simulink model "elec_linact_implementation"  (R2016a)
settings: Solver=ode23t  StartTime=0.0  StopTime=6  MaxStep=1e-2  RelTol=1e-3  AbsTol=1e-3
PostLoadFcn:
  | pwm_choice=1; % Variant control variable for PWM & H-Bridge subsystem
libraries: fl_lib x109, ee_lib x35, nesl_utility x16, fl_ps_legacy_lib x1, simulink x1
(part 1 of 2)
Description:
  | Linear Electric Actuator (Implementation Model)
  | 
  | This example shows a detailed implementation model of a controlled linear
  | actuator. The actuator consists of a DC motor driving a worm gear which in
  | turn drives a lead screw to produce linear motion. The model includes
  | quantization effects of the Hall-effect sensor and the implementation of the
  | control in analog electronics. Optionally, the PWM switching waveforms of
  | the PWM & H-Bridge subsystem can be included by right clicking on the
  | block and selecting Variant->Override using->pwm_choice==2. To simulate
  | with the actual semiconductor switching devices, select Variant->Override
  | using->pwm_choice==3. The model will run slowly with these options due
  | to the 10kHz switching and/or added component detail, but is useful for
  | validation of the system-averaged mode.
  | 
  | 
  | 
  | 
  | 
  | 
  | Copyright 2008-2016 The MathWorks, Inc.
settings Model: FPTRunName=Active  ExtModeAutoUpdateStatusClock=off  Creator=MathWorks  LastModifiedBy=Alireza
settings SolverCC: MaxConsecutiveMinStep=250  ZeroCrossControl=EnableAll
settings DataIOCC: LimitDataPoints=on  SaveFormat=Array  SignalLoggingSaveFormat=ModelDataLogs
settings OptimizationCC: ExpressionDepthLimit=2147483647  InitFltsAndDblsToZero=on
settings DebuggingCC: SaveWithParameterizedLinksMsg=none  UnderspecifiedInitializationDetection=Classic  MergeDetectMultiDrivingBlocksExec=none  SignalResolutionControl=TryResolveAllWithWarning  SolverPrmCheckMsg=warning  FcnCallInpInsideContextMsg=EnableAllAsWarning  StateNameClashWarn=warning
settings HardwareCC: ProdBitPerPointer=32  ProdLargestAtomicFloat=None  ProdIntDivRoundTo=Undefined  ProdEndianess=Unspecified  ProdWordSize=32  ProdHWDeviceType=32-bit Generic
settings ModelReferenceCC: PropagateSignalLabelsOutOfModel=off
settings GRTTargetCC: TargetFcnLib=ansi_tfl_tmw.mat  CombineOutputUpdateFcns=off  GRTInterface=on
settings ConfigComp: CovSFcnEnable=off
settings SimscapeCC: SimscapeNormalizeSystem=off

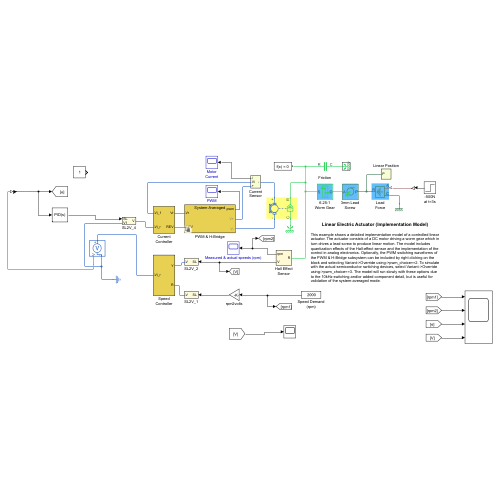
[thumbnail: Simulink's stored preview of the top-level diagram]
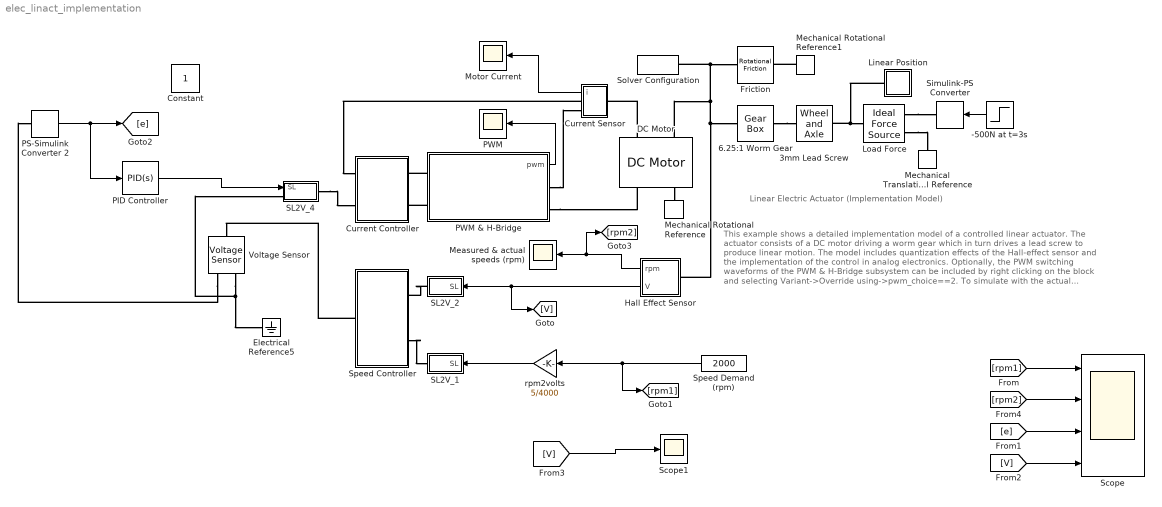
== system elec_linact_implementation ==
  note: Linear Electric Actuator (Implementation Model)
  note: This example shows a detailed implementation model of a controlled linear
      | actuator. The actuator consists of a DC motor driving a worm gear which in
      | turn drives a lead screw to produce linear motion. The model includes
      | quantization effects of the Hall-effect sensor and the implementation of the
      | control in analog electronics. Optionally, the PWM switching waveforms of
      | the PWM & H-Bridge subsystem can be included by right clicking on the
      | block and selecting Variant->Override using->pwm_choice==2. To simulate
      | with the actual semiconductor switching devices, select Variant->Override
      | using->pwm_choice==3. The model will run slowly with these options due
      | to the 10kHz switching and/or added component detail, but is useful for
      | validation of the system-averaged mode.
  -500N at t=3s : Step  Time=3  After=0  SampleTime=0
  3mm Lead Screw : fl_lib/Mechanical/Mechanisms/Wheel and Axle  R=3e-3/(2*pi) m  or=1  t_specify=off  t_priority=High  t=0 N*m  t_nominal_specify=off  t_nominal_unit=N*m  t_nominal_value=1  f_specify=off  f_priority=High  f=0 N  f_nominal_specify=off  f_nominal_unit=N  f_nominal_value=1
  6.25:1 Worm Gear : fl_lib/Mechanical/Mechanisms/Gear Box  ratio=6.25  t_in_specify=off  t_in_priority=High  t_in=0 N*m  t_in_nominal_specify=off  t_in_nominal_unit=N*m  t_in_nominal_value=1  t_out_specify=off  t_out_priority=High  t_out=0 N*m  t_out_nominal_specify=off  t_out_nominal_unit=N*m  t_out_nominal_value=1
  Constant : Constant
  Current Controller : Subsystem
  Current Sensor : Subsystem
  DC Motor : ee_lib/Electromechanical/Brushed Motors/DC Motor  field_option=ee.enum.field_option.pm  Rf=100 Ohm  Lf=1 H  Laf=0.15 H  If0=0 A  parameterization=1  Ra=4.8 Ohm  La=1600e-6 H  emf_or_torque=2  Kv=0.0637 V/rpm  Ki=0.066 N*m/A  T_stall=3e-3*4000/(2*pi*6.25) N*m  w_max=3250 rpm  w_rated=2375 rpm  P_rated=19 W  V_rated=24 V  lam_param=1  i_noload=0 A  V_i_noload=1.5 V  J=2.5e-5 kg*m^2  lam=1e-08 N*m/(rad/s)  speed0=0 rpm  enable_fault_armature=simscape.enum.onoff.off  rev_faulted=1 / 3  G_faulted_armature=1e-5 S  fault_trigger_armature=ee.enum.faults.faultTrigger.temporal  t_fault_armature=1 s  max_permissible_current_armature=inf A  t_fail_on_current_armature=1 s  enable_fault_field=simscape.enum.onoff.off  G_faulted_field=1e-5 S  fault_trigger_field=ee.enum.faults.faultTrigger.temporal  t_fault_field=1 s  max_permissible_current_field=inf A  t_fail_on_current_field=1 s  fault_action=simscape.enum.assert.action.none  alpha=3.93e-3 1/K  Tmeas=25 degC  thermal_mass=100 J/K  initial_temperature=25 degC
  Electrical Reference5 : fl_lib/Electrical/Electrical Elements/Electrical Reference
  Friction : fl_lib/Mechanical/Rotational Elements/Rotational Friction  brkwy_trq=0.022 N*m  brkwy_vel=0.03347 rad/s  Col_trq=0.022 N*m  visc_coef=0 N*m/(rad/s)  w_specify=off  w_priority=High  w=0 rad/s  w_nominal_specify=off  w_nominal_unit=rad/s  w_nominal_value=1  t_specify=off  t_priority=High  t=0 N*m  t_nominal_specify=off  t_nominal_unit=N*m  t_nominal_value=1
  Hall Effect Sensor : Subsystem
  Linear Position : Subsystem
  Load Force : fl_lib/Mechanical/Mechanical Sources/Ideal Force Source
  Measured & actual speeds (rpm) : Scope
  Mechanical Rotational Reference : fl_lib/Mechanical/Rotational Elements/Mechanical Rotational Reference
  Mechanical Rotational Reference1 : fl_lib/Mechanical/Rotational Elements/Mechanical Rotational Reference
  Mechanical Translational Reference : fl_lib/Mechanical/Translational Elements/Mechanical Translational Reference
  Motor Current : Scope
  PID Controller : simulink/Continuous/PID Controller  Controller=PID  Form=Parallel  TimeDomain=Continuous-time  SampleTime=-1  IntegratorMethod=Forward Euler  ControllerParametersSource=internal  P=1.8  I=18  D=0  N=100  UseFilter=on  InitialConditionSource=internal  InitialConditionForIntegrator=0  InitialConditionForFilter=0  DifferentiatorICPrevScaledInput=0  ExternalReset=none  TrackingMode=off  Kt=1  LimitOutput=off  UpperSaturationLimit=inf  LowerSaturationLimit=-inf  LinearizeAsGain=on  AntiWindupMode=none  Kb=1  POutMin=[]  POutMax=[]  IOutMin=[]  IOutMax=[]  DOutMin=[]  DOutMax=[]  NOutMin=[]  NOutMax=[]  SumOutMin=[]  SumOutMax=[]  SaturationOutMin=[]  SaturationOutMax=[]  PParamMin=[]  PParamMax=[]  IParamMin=[]  IParamMax=[]  DParamMin=[]  DParamMax=[]  NParamMin=[]  NParamMax=[]  KbParamMin=[]  KbParamMax=[]  KtParamMin=[]  KtParamMax=[]  KbOutMin=[]  KbOutMax=[]  KtOutMin=[]  KtOutMax=[]  IntegratorOutMin=[]  IntegratorOutMax=[]  FilterOutMin=[]  FilterOutMax=[]  SumI1OutMin=[]  SumI1OutMax=[]  SumI2OutMin=[]  SumI2OutMax=[]  SumI3OutMin=[]  SumI3OutMax=[]  SumDOutMin=[]  SumDOutMax=[]  DifferentiatorOutMin=[]  DifferentiatorOutMax=[]  IntegratorContinuousStateAttributes=''  IntegratorStateMustResolveToSignalObject=off  IntegratorRTWStateStorageClass=Auto  FilterContinuousStateAttributes=''  FilterStateMustResolveToSignalObject=off  FilterRTWStateStorageClass=Auto
  PS-Simulink Converter 2 : nesl_utility/PS-Simulink Converter  PhysicalDomain=network_engine_domain  SubClassName=ps_output  LeftPortType=input  RightPortType=output  PseudoPeriodic=off  Frequencies=[]  VectorFormat=1-D array  Unit=V  AffineConversion=off
  PWM : Scope
  PWM & H-Bridge : Subsystem  Variant=on  OverrideUsingVariant=pwm_choice==1
      settings: AttributesFormatString=%<BlockChoice>
  SL2V_1 : Subsystem
  SL2V_2 : Subsystem
  SL2V_4 : Subsystem
  Scope : Scope  NumInputPorts=4
  Scope1 : Scope
  Simulink-PS Converter : nesl_utility/Simulink-PS Converter  PhysicalDomain=network_engine_domain  SubClassName=ps_input  LeftPortType=input  RightPortType=output  PseudoPeriodic=off  Frequencies=[]  NoiseDistribution=none  NoiseParameters=[]  Unit=N  AffineConversion=off  FilteringAndDerivatives=zero  SimscapeFilterOrder=1  InputFilterTimeConstant=.001  UdotUserProvided=0
  Solver Configuration : nesl_utility/Solver Configuration  PhysicalDomain=network_engine_domain  SubClassName=solver  LeftPortType=input  RightPortType=generic  Tones=[]  Harmonics=[]  SimulateNoise=off  Profile=off  UseLocalSampling=off  EnableSwitchedLinearOptims=on  FrequencyDomain=off  UseCCode=off  RelTol=0.001  AbsTol=1e-06  MinStep=1e-09  ToWorkspace=off  RevertToSquareIcSolve=off  NumHomotopyIterations=100  PhasorMode=off  PhasorModeNumHarmonics=1  IndexReductionMethod=DerivativeReplacement  DoDC=off  ResidualTolerance=1e-9  UseLocalSolver=off  LocalSolverChoice=NE_BACKWARD_EULER_ADVANCER  LocalSolverSampleTime=.001  DoFixedCost=off  MaxNonlinIter=3  MaxModeIter=2  ComputeImpulses=off  ImpulseIterations=2  LinearAlgebra=Sparse  LinearAlgebraNumThread=0  EquationFormulation=NE_TIME_EF  DelaysMemoryBudget=1024  AutomaticFiltering=on  FilteringTimeConstant=0.001  PartitionStorageMethod=AS_NEEDED  PartitionMemoryBudget=1024  PartitionMethod=FAST
  Speed Controller : Subsystem
  Speed Demand (rpm) : Constant  Value=2000
  Voltage Sensor : fl_lib/Electrical/Electrical Sensors/Voltage Sensor
  rpm2volts : Gain  Gain=5/4000
  wires:
  -500N at t=3s/1 -> Simulink-PS Converter/1
  rpm2volts/1 -> SL2V_1/1(SL)
  Hall Effect Sensor/2(V) -> [V], SL2V_2/1(SL)
  Hall Effect Sensor/1(rpm) -> [rpm2], Measured & actual speeds (rpm)/1
  Current Sensor/1(i) -> Motor Current/1
  PWM & H-Bridge/1(pwm) -> PWM/1
  PID Controller/1 -> SL2V_4/1(SL)
  PS-Simulink Converter 2/1 -> [e], PID Controller/1
  Speed Demand (rpm)/1 -> rpm2volts/1, [rpm1]
  [rpm1] -> Scope/1
  [rpm2] -> Scope/2
  [e] -> Scope/3
  [V] -> Scope/4
  [V] -> Scope1/1
  connections:
  DC Motor/RConn2 -- Mechanical Rotational Reference/LConn1
  6.25:1 Worm Gear/RConn1 -- 3mm Lead Screw/LConn1
  Linear Position/LConn1 -- Load Force/LConn1 -- 3mm Lead Screw/RConn1
  Load Force/RConn2 -- Mechanical Translational Reference/LConn1
  Load Force/RConn1 -- Simulink-PS Converter/RConn1
  Hall Effect Sensor/LConn1 -- DC Motor/LConn2 -- Solver Configuration/RConn1 -- Friction/LConn1 -- 6.25:1 Worm Gear/LConn1
  PWM & H-Bridge/RConn1 -- Current Sensor/RConn2
  DC Motor/LConn1 -- Current Sensor/LConn1
  PWM & H-Bridge/LConn1 -- Current Controller/RConn1
  PWM & H-Bridge/LConn2 -- Current Controller/RConn2
  Mechanical Rotational Reference1/LConn1 -- Friction/RConn1
  Speed Controller/LConn2 -- SL2V_1/RConn1
  Current Sensor/RConn1 -- Current Controller/LConn1
  SL2V_2/RConn1 -- Speed Controller/LConn1
  PWM & H-Bridge/RConn2 -- DC Motor/RConn1
  Voltage Sensor/RConn2 -- SL2V_4/LConn1 -- Electrical Reference5/LConn1
  Speed Controller/RConn1 -- Voltage Sensor/LConn1
  SL2V_4/RConn1 -- Current Controller/LConn2
  Voltage Sensor/RConn1 -- PS-Simulink Converter 2/LConn1

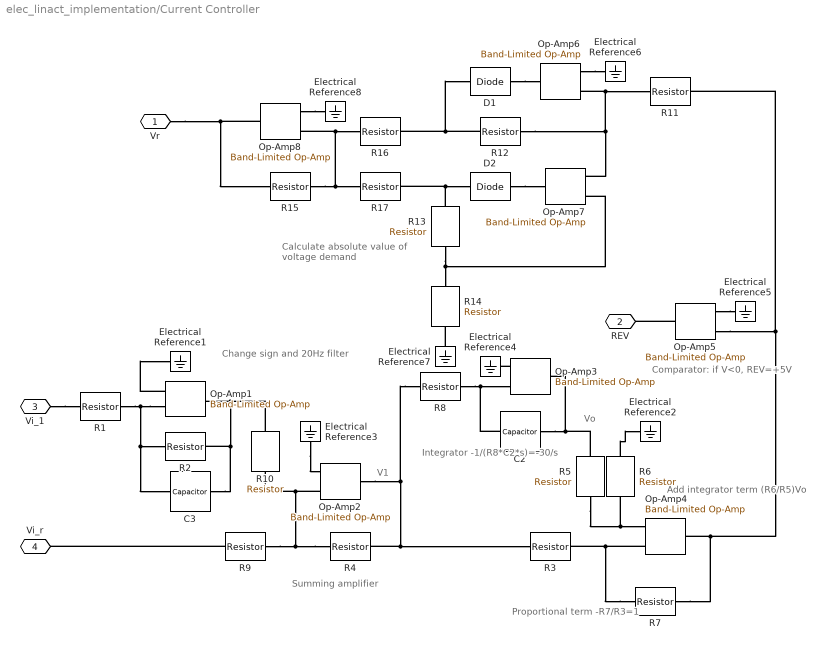
== system elec_linact_implementation/Current Controller ==
  note: Summing
      | amplifier
  note: Integrator
      | -1/(R8*C2*s)=-30/s
  note: Proportional
      | term -R7/R3=1
  note: Add integrator
      | term (R6/R5)Vo
  note: Vo
  note: V1
  note: Change sign
      | and 20Hz filter
  note: Comparator: if
      | V<0, REV=+5V
  note: Calculate absolute value
      | of voltage demand
  C2 : fl_lib/Electrical/Electrical Elements/Capacitor  c=10 uF  r=0.1 Ohm  g=0 1/Ohm  i_specify=off  i_priority=High  i=0 A  i_nominal_specify=off  i_nominal_unit=A  i_nominal_value=1  v_specify=off  v_priority=High  v=0 V  v_nominal_specify=off  v_nominal_unit=V  v_nominal_value=1  vc_specify=on  vc_priority=High  vc=0 V  vc_nominal_specify=off  vc_nominal_unit=V  vc_nominal_value=1
  C3 : fl_lib/Electrical/Electrical Elements/Capacitor  c=0.8 uF  r=0.1 Ohm  g=0 1/Ohm  i_specify=off  i_priority=High  i=0 A  i_nominal_specify=off  i_nominal_unit=A  i_nominal_value=1  v_specify=off  v_priority=High  v=0 V  v_nominal_specify=off  v_nominal_unit=V  v_nominal_value=1  vc_specify=on  vc_priority=High  vc=0 V  vc_nominal_specify=off  vc_nominal_unit=V  vc_nominal_value=1
  D1 : ee_lib/Semiconductors & Converters/Diode  ModelType=ee.enum.diode.modelType.pwl  TableType=ee.enum.diode.tableType.IfMat  IfMat=[.07, .12, .19, 1.75, 4.24, 7.32, 11.2; .16, .3, .72, 2.14, 5.02, 8.35, 13.12] A  VfMat=[.9, 1.15, 1.25, 1.5, 1.75, 2.17, 2.6, 2.85; .58, .68, .75, 1.1, 1.38, 1.77, 2.27, 2.7] V  TjVec=[25, 125] degC  VfVec=[.5, .7, .9, 1.3, 1.7, 2.1, 2.5] V  IfVec=[.1, .2, .5, 1, 2, 4, 7, 10] A  Vf=0.6 V  Ron=0.3 Ohm  Goff=1e-08 1/Ohm  prmExp=1  I12="[  0.07 1.5 ] A"  V12="[  0.7 0.8 ] V"  RS=0 Ohm  Tmeas=298.15 K  IS=1e-14 A  ec=1  I1=0.0137 A  V1=0.6 V  N_series=1  N_parallel=1  Rz=0.3 Ohm  BV=inf V  C_param=1  CJ=5 pF  CJ0=50 pF  Vvec="[  0.1 10 100 ] V"  Cvec="[  3.5 1 0.4 ] pF"  VJ=1 V  Mgrad=0.5  FC=0.5  Q_param=ee.enum.diode.recoveryParam.off  iRM=-7.15 A  iF=4 A  didt=-750 A/us  trr_factor=3  trr=115 ns  Qrr=1500 s*uA  Vr=-600 V  Ls=150 nH  Erec=0.03 J  TT=50 ns  tau=100 ns  T_param=1  Tdevice=25 degC  I1_T2=0.245 A  V1_T2=0.5 V  IS_T2=1.25e-7 A  Tmeas2=125 degC  XTI_param=1  XTI=3  EG_param=1  EG=1.11 eV  dBVdT=0 V/K  enable_faults=simscape.enum.onoff.off  fault_action=simscape.enum.assert.action.none  fault_types=ee.enum.diode.faults.open  tau_fault=1e-3 s  IfMat_faulted=[.07, .12, .19, 1.75, 4.24, 7.32, 11.2; .16, .3, .72, 2.14, 4.02, 6.35, 9.12] A  VfMat_faulted=[.9, 1.15, 1.25, 1.5, 1.75, 2.17, 2.6, 2.85; .58, .68, .75, 1.1, 1.38, 1.77, 2.27, 2.7] V  VfVec_faulted=[.5, .7, .9, 1.3, 1.7, 2.1, 2.5] V  IfVec_faulted=[.1, .2, .5, 1, 2, 4, 7, 10] A  Ropen_faulted=1000 Ohm  Gshort_faulted=1000 1/Ohm  Vf_faulted=0.6 V  Ron_faulted=0.3 Ohm  Goff_faulted=1e-8 S  I12_faulted=[.0137, .545] A  V12_faulted=[.6, .7] V  IS_faulted=1e-12 A  ec_faulted=1  I1_faulted=0.0137 A  V1_faulted=0.6 V  RS_faulted=0 Ohm  Rz_faulted=0.3 Ohm  BV_faulted=inf V  Cscale_faulted=100  enable_temporal_fault=simscape.enum.onoff.off  t_fault=inf s  enable_behavioral_fault=simscape.enum.onoff.off  max_permissible_voltage=inf V  n_fail_on_voltage=1  max_permissible_current=inf A  t_fail_on_current=1 s  max_permissible_dVdt=inf V/s  enable_fault_input=simscape.enum.onoff.off  i_specify=off  i_priority=None  i=0 A  i_nominal_specify=off  i_nominal_unit=A  i_nominal_value=1  v_specify=off  v_priority=None  v=0 V  v_nominal_specify=off  v_nominal_unit=V  v_nominal_value=1  i_diode_specify=off  i_diode_priority=None  i_diode=0 A  i_diode_nominal_specify=off  i_diode_nominal_unit=A  i_diode_nominal_value=1  v_diode_specify=off  v_diode_priority=None  v_diode=0 V  v_diode_nominal_specify=off  v_diode_nominal_unit=V  v_diode_nominal_value=1  i_capacitor_specify=off  i_capacitor_priority=None  i_capacitor=0 A  i_capacitor_nominal_specify=off  i_capacitor_nominal_unit=A  i_capacitor_nominal_value=1  v_capacitor_specify=off  v_capacitor_priority=None  v_capacitor=0 V  v_capacitor_nominal_specify=off  v_capacitor_nominal_unit=V  v_capacitor_nominal_value=1  power_dissipated_specify=off  power_dissipated_priority=None  power_dissipated=0 W  power_dissipated_nominal_specify=off  power_dissipated_nominal_unit=W  power_dissipated_nominal_value=1  max_permissible_temperature=inf K  t_fail_on_temperature=1 s  thermal_network_parameterization=ee.enum.thermalNetworkTopology.junctionCase  Rth=[0, 10] K/W  Rth_Cauer=[1, 3, 10] K/W  Rth_Foster=[4, 6] K/W  thermal_mass_parameterization=ee.enum.thermalNetwork.timeconstant  thermal_mass=[0, 1] J/K  thermal_mass_Cauer=[.1, .3, 1] J/K  thermal_mass_Foster=[1.5, 3] J/K  thermal_time_constant=[0, 10] s  thermal_time_constant_Cauer=[1, 3, 10] s  thermal_time_constant_Foster=[6, 18] s  thermal_mass_initial_temperatures=[25, 25] degC  thermal_mass_initial_temperatures_Cauer=[25, 25, 25] degC  steadyState_Foster=simscape.enum.onoff.on  Tvec_initial_Foster=[25, 25, 25, 25] degC
  D2 : ee_lib/Semiconductors & Converters/Diode  ModelType=ee.enum.diode.modelType.pwl  TableType=ee.enum.diode.tableType.IfMat  IfMat=[.07, .12, .19, 1.75, 4.24, 7.32, 11.2; .16, .3, .72, 2.14, 5.02, 8.35, 13.12] A  VfMat=[.9, 1.15, 1.25, 1.5, 1.75, 2.17, 2.6, 2.85; .58, .68, .75, 1.1, 1.38, 1.77, 2.27, 2.7] V  TjVec=[25, 125] degC  VfVec=[.5, .7, .9, 1.3, 1.7, 2.1, 2.5] V  IfVec=[.1, .2, .5, 1, 2, 4, 7, 10] A  Vf=0.6 V  Ron=0.3 Ohm  Goff=1e-08 1/Ohm  prmExp=1  I12="[  0.07 1.5 ] A"  V12="[  0.7 0.8 ] V"  RS=0 Ohm  Tmeas=298.15 K  IS=1e-14 A  ec=1  I1=0.0137 A  V1=0.6 V  N_series=1  N_parallel=1  Rz=0.3 Ohm  BV=inf V  C_param=1  CJ=5 pF  CJ0=50 pF  Vvec="[  0.1 10 100 ] V"  Cvec="[  3.5 1 0.4 ] pF"  VJ=1 V  Mgrad=0.5  FC=0.5  Q_param=ee.enum.diode.recoveryParam.off  iRM=-7.15 A  iF=4 A  didt=-750 A/us  trr_factor=3  trr=115 ns  Qrr=1500 s*uA  Vr=-600 V  Ls=150 nH  Erec=0.03 J  TT=50 ns  tau=100 ns  T_param=1  Tdevice=25 degC  I1_T2=0.245 A  V1_T2=0.5 V  IS_T2=1.25e-7 A  Tmeas2=125 degC  XTI_param=1  XTI=3  EG_param=1  EG=1.11 eV  dBVdT=0 V/K  enable_faults=simscape.enum.onoff.off  fault_action=simscape.enum.assert.action.none  fault_types=ee.enum.diode.faults.open  tau_fault=1e-3 s  IfMat_faulted=[.07, .12, .19, 1.75, 4.24, 7.32, 11.2; .16, .3, .72, 2.14, 4.02, 6.35, 9.12] A  VfMat_faulted=[.9, 1.15, 1.25, 1.5, 1.75, 2.17, 2.6, 2.85; .58, .68, .75, 1.1, 1.38, 1.77, 2.27, 2.7] V  VfVec_faulted=[.5, .7, .9, 1.3, 1.7, 2.1, 2.5] V  IfVec_faulted=[.1, .2, .5, 1, 2, 4, 7, 10] A  Ropen_faulted=1000 Ohm  Gshort_faulted=1000 1/Ohm  Vf_faulted=0.6 V  Ron_faulted=0.3 Ohm  Goff_faulted=1e-8 S  I12_faulted=[.0137, .545] A  V12_faulted=[.6, .7] V  IS_faulted=1e-12 A  ec_faulted=1  I1_faulted=0.0137 A  V1_faulted=0.6 V  RS_faulted=0 Ohm  Rz_faulted=0.3 Ohm  BV_faulted=inf V  Cscale_faulted=100  enable_temporal_fault=simscape.enum.onoff.off  t_fault=inf s  enable_behavioral_fault=simscape.enum.onoff.off  max_permissible_voltage=inf V  n_fail_on_voltage=1  max_permissible_current=inf A  t_fail_on_current=1 s  max_permissible_dVdt=inf V/s  enable_fault_input=simscape.enum.onoff.off  i_specify=off  i_priority=None  i=0 A  i_nominal_specify=off  i_nominal_unit=A  i_nominal_value=1  v_specify=off  v_priority=None  v=0 V  v_nominal_specify=off  v_nominal_unit=V  v_nominal_value=1  i_diode_specify=off  i_diode_priority=None  i_diode=0 A  i_diode_nominal_specify=off  i_diode_nominal_unit=A  i_diode_nominal_value=1  v_diode_specify=off  v_diode_priority=None  v_diode=0 V  v_diode_nominal_specify=off  v_diode_nominal_unit=V  v_diode_nominal_value=1  i_capacitor_specify=off  i_capacitor_priority=None  i_capacitor=0 A  i_capacitor_nominal_specify=off  i_capacitor_nominal_unit=A  i_capacitor_nominal_value=1  v_capacitor_specify=off  v_capacitor_priority=None  v_capacitor=0 V  v_capacitor_nominal_specify=off  v_capacitor_nominal_unit=V  v_capacitor_nominal_value=1  power_dissipated_specify=off  power_dissipated_priority=None  power_dissipated=0 W  power_dissipated_nominal_specify=off  power_dissipated_nominal_unit=W  power_dissipated_nominal_value=1  max_permissible_temperature=inf K  t_fail_on_temperature=1 s  thermal_network_parameterization=ee.enum.thermalNetworkTopology.junctionCase  Rth=[0, 10] K/W  Rth_Cauer=[1, 3, 10] K/W  Rth_Foster=[4, 6] K/W  thermal_mass_parameterization=ee.enum.thermalNetwork.timeconstant  thermal_mass=[0, 1] J/K  thermal_mass_Cauer=[.1, .3, 1] J/K  thermal_mass_Foster=[1.5, 3] J/K  thermal_time_constant=[0, 10] s  thermal_time_constant_Cauer=[1, 3, 10] s  thermal_time_constant_Foster=[6, 18] s  thermal_mass_initial_temperatures=[25, 25] degC  thermal_mass_initial_temperatures_Cauer=[25, 25, 25] degC  steadyState_Foster=simscape.enum.onoff.on  Tvec_initial_Foster=[25, 25, 25, 25] degC
  Electrical Reference{1..8} (8 alike) : fl_lib/Electrical/Electrical Elements/Electrical Reference
  Op-Amp{1..8} (8 alike) : ee_lib/Integrated Circuits/Band-Limited Op-Amp  A=1000  Rin=1e+06 Ohm  Rout=100 Ohm  Vmin=-5 V  Vmax=5 V  Vdotmax=1000 V/s  f=1e3 Hz  V0=0 V
  R{1..7,9..17} (16 alike) : fl_lib/Electrical/Electrical Elements/Resistor  R=10 kOhm  i_specify=off  i_priority=High  i=0 A  i_nominal_specify=off  i_nominal_unit=A  i_nominal_value=1  v_specify=off  v_priority=High  v=0 V  v_nominal_specify=off  v_nominal_unit=V  v_nominal_value=1
  R8 : fl_lib/Electrical/Electrical Elements/Resistor  R=3.3 kOhm  i_specify=off  i_priority=High  i=0 A  i_nominal_specify=off  i_nominal_unit=A  i_nominal_value=1  v_specify=off  v_priority=High  v=0 V  v_nominal_specify=off  v_nominal_unit=V  v_nominal_value=1
  Vr : PMIOPort  Side=Right
  REV : PMIOPort  Port=2  Side=Right
  Vi_1 : PMIOPort  Port=3  Side=Left
  Vi_r : PMIOPort  Port=4  Side=Left
  connections:
  R9/LConn1 -- Vi_r/RConn1
  R8/LConn1 -- Op-Amp2/RConn1 -- R3/LConn1 -- R4/RConn1
  R8/RConn1 -- Op-Amp3/LConn2 -- C2/LConn1
  R5/LConn1 -- Op-Amp3/RConn1 -- C2/RConn1
  Op-Amp5/LConn2 -- R11/RConn1 -- R7/RConn1 -- Op-Amp4/RConn1
  R6/LConn1 -- Op-Amp4/LConn1 -- R5/RConn1
  R7/LConn1 -- Op-Amp4/LConn2 -- R3/RConn1
  R4/LConn1 -- Op-Amp2/LConn2 -- R10/RConn1 -- R9/RConn1
  Op-Amp1/LConn2 -- R2/LConn1 -- C3/LConn1 -- R1/RConn1
  Op-Amp1/RConn1 -- R2/RConn1 -- C3/RConn1 -- R10/LConn1
  Op-Amp1/LConn1 -- Electrical Reference1/LConn1
  Op-Amp3/LConn1 -- Electrical Reference4/LConn1
  Electrical Reference3/LConn1 -- Op-Amp2/LConn1
  R6/RConn1 -- Electrical Reference2/LConn1
  Vi_1/RConn1 -- R1/LConn1
  Op-Amp5/LConn1 -- Electrical Reference5/LConn1
  Op-Amp5/RConn1 -- REV/RConn1
  R12/RConn1 -- Op-Amp6/LConn2 -- R11/LConn1 -- Op-Amp7/LConn1
  Op-Amp6/LConn1 -- Electrical Reference6/LConn1
  R13/RConn1 -- R14/LConn1 -- Op-Amp7/LConn2
  Electrical Reference7/LConn1 -- R14/RConn1
  D1/RConn1 -- Op-Amp6/RConn1
  R12/LConn1 -- D1/LConn1 -- R16/RConn1
  D2/RConn1 -- Op-Amp7/RConn1
  R13/LConn1 -- D2/LConn1 -- R17/RConn1
  Vr/RConn1 -- Op-Amp8/RConn1 -- R15/LConn1
  R15/RConn1 -- Op-Amp8/LConn2 -- R16/LConn1 -- R17/LConn1
  Op-Amp8/LConn1 -- Electrical Reference8/LConn1

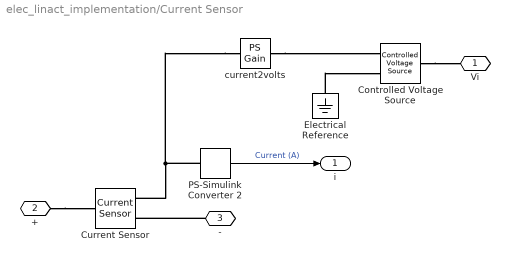
== system elec_linact_implementation/Current Sensor ==
  Controlled Voltage Source : fl_lib/Electrical/Electrical Sources/Controlled Voltage Source
  Current Sensor : fl_lib/Electrical/Electrical Sensors/Current Sensor
  Electrical Reference : fl_lib/Electrical/Electrical Elements/Electrical Reference
  PS-Simulink Converter 2 : nesl_utility/PS-Simulink Converter  PhysicalDomain=network_engine_domain  SubClassName=ps_output  LeftPortType=input  RightPortType=output  PseudoPeriodic=off  Frequencies=[]  VectorFormat=1-D array  Unit=A  AffineConversion=off
  current2volts : fl_ps_legacy_lib/Legacy Physical Signals/Functions/PS Gain  gain=1
  Vi : PMIOPort  Side=Right
  + : PMIOPort  Port=2  Side=Right
  - : PMIOPort  Port=3  Side=Left
  i : Outport
  wires:
  PS-Simulink Converter 2/1 -> i/1  "Current (A)"
  connections:
  +/RConn1 -- Current Sensor/LConn1
  -/RConn1 -- Current Sensor/RConn2
  current2volts/LConn1 -- PS-Simulink Converter 2/LConn1 -- Current Sensor/RConn1
  Electrical Reference/LConn1 -- Controlled Voltage Source/RConn2
  Controlled Voltage Source/LConn1 -- Vi/RConn1
  current2volts/RConn1 -- Controlled Voltage Source/RConn1

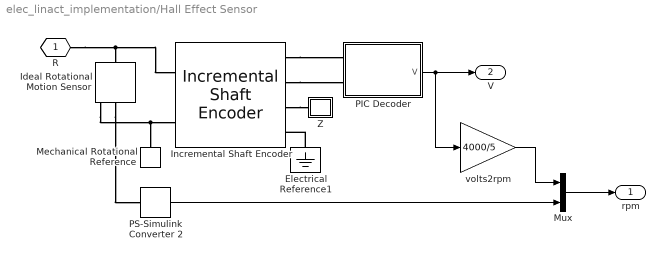
== system elec_linact_implementation/Hall Effect Sensor ==
  Electrical Reference1 : fl_lib/Electrical/Electrical Elements/Electrical Reference
  Ideal Rotational Motion Sensor : fl_lib/Mechanical/Mechanical Sensors/Ideal Rotational Motion Sensor  wrap_angle=simscape.enum.onoff.off  offset=0 rad
  Incremental Shaft Encoder : ee_lib/Sensors & Transducers/Incremental Shaft Encoder  NPulse=2  Vm=5 V  angle0=0 deg
      settings: InternalSimscapePortConfiguration="{\"Bottom\":[],\"Left\":[{\"id\":\"R\",\"label\":\"R\",\"type\":\"foundation.mechanical.rotational.rotational\"},{\"id\":\"C\",\"label\":\"C\",\"type\":\"foundation.mechanical.rotational.rotational\"}],\"Right\":[{\"id\":\"A\",\"label\":\"A\",\"type\":\"foundation.electrical.electrical\"},{\"id\":\"B\",\"label\":\"B\",\"type\":\"foundation.electrical.electrical\"},{\"id\":\"Z\",\"label\":\"Z\",\"type\":\"foundation.electrical.electrical\"},{\"id\":\"GND\",\"label\":\"REF\",\"type\":\"foundation.electrical.electrical\"}],\"Top\":[]}"
  Mechanical Rotational Reference : fl_lib/Mechanical/Rotational Elements/Mechanical Rotational Reference
  Mux : Mux  Inputs=2
  PIC Decoder : Subsystem
  PS-Simulink Converter 2 : nesl_utility/PS-Simulink Converter  PhysicalDomain=network_engine_domain  SubClassName=ps_output  LeftPortType=input  RightPortType=output  PseudoPeriodic=off  Frequencies=[]  VectorFormat=1-D array  Unit=rpm  AffineConversion=off
  Z : Subsystem
  volts2rpm : Gain  Gain=4000/5
  R : PMIOPort  Side=Left
  rpm : Outport
  V : Outport  Port=2
  wires:
  PS-Simulink Converter 2/1 -> Mux/2
  Mux/1 -> rpm/1
  PIC Decoder/1(V) -> volts2rpm/1, V/1
  volts2rpm/1 -> Mux/1
  connections:
  Ideal Rotational Motion Sensor/RConn2 -- PS-Simulink Converter 2/LConn1
  Ideal Rotational Motion Sensor/RConn1 -- Incremental Shaft Encoder/LConn2 -- Mechanical Rotational Reference/LConn1
  R/RConn1 -- Ideal Rotational Motion Sensor/LConn1 -- Incremental Shaft Encoder/LConn1
  Electrical Reference1/LConn1 -- Incremental Shaft Encoder/RConn4
  Incremental Shaft Encoder/RConn3 -- Z/LConn1
  Incremental Shaft Encoder/RConn1 -- PIC Decoder/LConn1
  Incremental Shaft Encoder/RConn2 -- PIC Decoder/LConn2

== system elec_linact_implementation/Linear Position ==
  Linear Position (mm) : Scope
  Linear Speed (mm/s) : Scope
  Mechanical Translational Reference : fl_lib/Mechanical/Translational Elements/Mechanical Translational Reference
  PS-Simulink Converter 1 : nesl_utility/PS-Simulink Converter  PhysicalDomain=network_engine_domain  SubClassName=ps_output  LeftPortType=input  RightPortType=output  PseudoPeriodic=off  Frequencies=[]  VectorFormat=1-D array  Unit=mm/s  AffineConversion=off
  PS-Simulink Converter 3 : nesl_utility/PS-Simulink Converter  PhysicalDomain=network_engine_domain  SubClassName=ps_output  LeftPortType=input  RightPortType=output  PseudoPeriodic=off  Frequencies=[]  VectorFormat=1-D array  Unit=mm  AffineConversion=off
  Sensor1 : fl_lib/Mechanical/Mechanical Sensors/Ideal Translational Motion Sensor  offset=0 m
  P : PMIOPort  Side=Left
  wires:
  PS-Simulink Converter 3/1 -> Linear Position (mm)/1
  PS-Simulink Converter 1/1 -> Linear Speed (mm/s)/1
  connections:
  Sensor1/RConn1 -- Mechanical Translational Reference/LConn1
  Sensor1/RConn3 -- PS-Simulink Converter 3/LConn1
  P/RConn1 -- Sensor1/LConn1
  Sensor1/RConn2 -- PS-Simulink Converter 1/LConn1

== system elec_linact_implementation/PWM & H-Bridge ==
  Implementation : Subsystem  VariantControl=pwm_choice==3
  System-Averaged : Subsystem  VariantControl=pwm_choice==1
  System-PWM : Subsystem  VariantControl=pwm_choice==2
  Vr : PMIOPort  Side=Left
  REV : PMIOPort  Port=2  Side=Left
  V+ : PMIOPort  Port=3  Side=Right
  V- : PMIOPort  Port=4  Side=Right
  pwm : Outport

== system elec_linact_implementation/SL2V_1 ==
  SL : Inport
  Controlled Voltage Source : fl_lib/Electrical/Electrical Sources/Controlled Voltage Source
  Electrical Reference : fl_lib/Electrical/Electrical Elements/Electrical Reference
  Simulink-PS Converter : nesl_utility/Simulink-PS Converter  PhysicalDomain=network_engine_domain  SubClassName=ps_input  LeftPortType=input  RightPortType=output  PseudoPeriodic=off  Frequencies=[]  NoiseDistribution=none  NoiseParameters=[]  Unit=V  AffineConversion=off  FilteringAndDerivatives=zero  SimscapeFilterOrder=1  InputFilterTimeConstant=.001  UdotUserProvided=0
  V : PMIOPort  Side=Right
  wires:
  SL/1 -> Simulink-PS Converter/1
  connections:
  Electrical Reference/LConn1 -- Controlled Voltage Source/RConn2
  V/RConn1 -- Controlled Voltage Source/LConn1
  Simulink-PS Converter/RConn1 -- Controlled Voltage Source/RConn1

== system elec_linact_implementation/SL2V_2 ==
  SL : Inport
  Controlled Voltage Source : fl_lib/Electrical/Electrical Sources/Controlled Voltage Source
  Electrical Reference : fl_lib/Electrical/Electrical Elements/Electrical Reference
  Simulink-PS Converter : nesl_utility/Simulink-PS Converter  PhysicalDomain=network_engine_domain  SubClassName=ps_input  LeftPortType=input  RightPortType=output  PseudoPeriodic=off  Frequencies=[]  NoiseDistribution=none  NoiseParameters=[]  Unit=V  AffineConversion=off  FilteringAndDerivatives=zero  SimscapeFilterOrder=1  InputFilterTimeConstant=.001  UdotUserProvided=0
  V : PMIOPort  Side=Right
  wires:
  SL/1 -> Simulink-PS Converter/1
  connections:
  Simulink-PS Converter/RConn1 -- Controlled Voltage Source/RConn1
  V/RConn1 -- Controlled Voltage Source/LConn1
  Electrical Reference/LConn1 -- Controlled Voltage Source/RConn2

== system elec_linact_implementation/SL2V_4 ==
  SL : Inport
  Controlled Voltage Source : fl_lib/Electrical/Electrical Sources/Controlled Voltage Source
  Electrical Reference : fl_lib/Electrical/Electrical Elements/Electrical Reference
  Simulink-PS Converter : nesl_utility/Simulink-PS Converter  PhysicalDomain=network_engine_domain  SubClassName=ps_input  LeftPortType=input  RightPortType=output  PseudoPeriodic=off  Frequencies=[]  NoiseDistribution=none  NoiseParameters=[]  Unit=V  AffineConversion=off  FilteringAndDerivatives=zero  SimscapeFilterOrder=1  InputFilterTimeConstant=.001  UdotUserProvided=0
  V : PMIOPort  Side=Right
  V1 : PMIOPort  Port=2  Side=Left
  wires:
  SL/1 -> Simulink-PS Converter/1
  connections:
  Electrical Reference/LConn1 -- V1/RConn1 -- Controlled Voltage Source/RConn2
  V/RConn1 -- Controlled Voltage Source/LConn1
  Simulink-PS Converter/RConn1 -- Controlled Voltage Source/RConn1

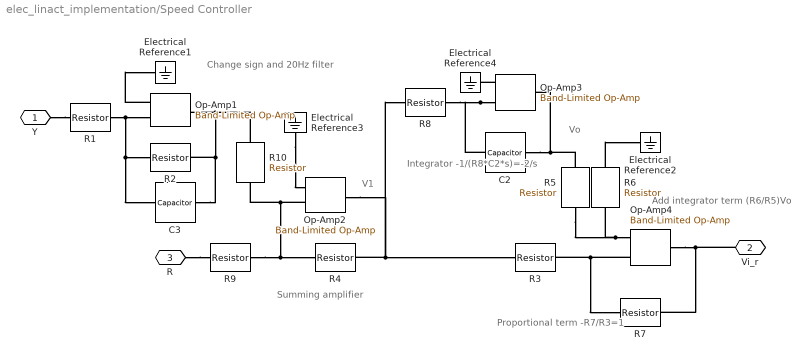
== system elec_linact_implementation/Speed Controller ==
  note: Summing
      | amplifier
  note: Integrator
      | -1/(R8*C2*s)=-2/s
  note: Proportional
      | term -R7/R3=1
  note: Add integrator
      | term (R6/R5)Vo
  note: Vo
  note: V1
  note: Change sign
      | and 20Hz filter
  C2 : fl_lib/Electrical/Electrical Elements/Capacitor  c=10 uF  r=0.1 Ohm  g=0 1/Ohm  i_specify=off  i_priority=High  i=0 A  i_nominal_specify=off  i_nominal_unit=A  i_nominal_value=1  v_specify=off  v_priority=High  v=0 V  v_nominal_specify=off  v_nominal_unit=V  v_nominal_value=1  vc_specify=on  vc_priority=High  vc=0 V  vc_nominal_specify=off  vc_nominal_unit=V  vc_nominal_value=1
  C3 : fl_lib/Electrical/Electrical Elements/Capacitor  c=0.8 uF  r=0.1 Ohm  g=0 1/Ohm  i_specify=off  i_priority=High  i=0 A  i_nominal_specify=off  i_nominal_unit=A  i_nominal_value=1  v_specify=off  v_priority=High  v=0 V  v_nominal_specify=off  v_nominal_unit=V  v_nominal_value=1  vc_specify=on  vc_priority=High  vc=0 V  vc_nominal_specify=off  vc_nominal_unit=V  vc_nominal_value=1
  Electrical Reference{1..4} (4 alike) : fl_lib/Electrical/Electrical Elements/Electrical Reference
  Op-Amp{1..4} (4 alike) : ee_lib/Integrated Circuits/Band-Limited Op-Amp  A=1000  Rin=1e+06 Ohm  Rout=100 Ohm  Vmin=-5 V  Vmax=5 V  Vdotmax=1000 V/s  f=1e3 Hz  V0=0 V
  R{1..7,9..10} (9 alike) : fl_lib/Electrical/Electrical Elements/Resistor  R=10 kOhm  i_specify=off  i_priority=High  i=0 A  i_nominal_specify=off  i_nominal_unit=A  i_nominal_value=1  v_specify=off  v_priority=High  v=0 V  v_nominal_specify=off  v_nominal_unit=V  v_nominal_value=1
  R8 : fl_lib/Electrical/Electrical Elements/Resistor  R=55 kOhm  i_specify=off  i_priority=High  i=0 A  i_nominal_specify=off  i_nominal_unit=A  i_nominal_value=1  v_specify=off  v_priority=High  v=0 V  v_nominal_specify=off  v_nominal_unit=V  v_nominal_value=1
  Y : PMIOPort  Side=Left
  Vi_r : PMIOPort  Port=2  Side=Right
  R : PMIOPort  Port=3  Side=Left
  connections:
  R8/LConn1 -- Op-Amp2/RConn1 -- R4/RConn1 -- R3/LConn1
  Op-Amp3/LConn2 -- R8/RConn1 -- C2/LConn1
  R5/LConn1 -- Op-Amp3/RConn1 -- C2/RConn1
  Op-Amp4/RConn1 -- Vi_r/RConn1 -- R7/RConn1
  Op-Amp4/LConn1 -- R6/LConn1 -- R5/RConn1
  Op-Amp4/LConn2 -- R7/LConn1 -- R3/RConn1
  Op-Amp2/LConn2 -- R10/RConn1 -- R4/LConn1 -- R9/RConn1
  R1/RConn1 -- Op-Amp1/LConn2 -- C3/LConn1 -- R2/LConn1
  R10/LConn1 -- Op-Amp1/RConn1 -- C3/RConn1 -- R2/RConn1
  Y/RConn1 -- R1/LConn1
  Electrical Reference3/LConn1 -- Op-Amp2/LConn1
  Op-Amp1/LConn1 -- Electrical Reference1/LConn1
  R/RConn1 -- R9/LConn1
  R6/RConn1 -- Electrical Reference2/LConn1
  Op-Amp3/LConn1 -- Electrical Reference4/LConn1

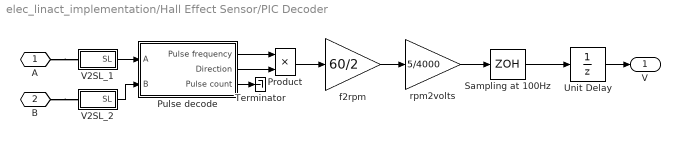
== system elec_linact_implementation/Hall Effect Sensor/PIC Decoder ==
  Product : Product  RndMeth=Zero
  Pulse decode : Subsystem
  Sampling at 100Hz : ZeroOrderHold  SampleTime=0.01
  Terminator : Terminator
  Unit Delay : UnitDelay  SampleTime=0.01  HasFrameUpgradeWarning=on
  V2SL_1 : Subsystem
  V2SL_2 : Subsystem
  f2rpm : Gain  Gain=60/2
  rpm2volts : Gain  Gain=5/4000
  A : PMIOPort  Side=Left
  B : PMIOPort  Port=2  Side=Left
  V : Outport
  wires:
  Product/1 -> f2rpm/1
  Pulse decode/2(Direction) -> Product/2
  Pulse decode/1(Pulse frequency) -> Product/1
  Pulse decode/3(Pulse count) -> Terminator/1
  f2rpm/1 -> rpm2volts/1
  rpm2volts/1 -> Sampling at 100Hz/1
  V2SL_1/1(SL) -> Pulse decode/1(A)
  V2SL_2/1(SL) -> Pulse decode/2(B)
  Sampling at 100Hz/1 -> Unit Delay/1
  Unit Delay/1 -> V/1
  connections:
  A/RConn1 -- V2SL_1/LConn1
  B/RConn1 -- V2SL_2/LConn1

== system elec_linact_implementation/Hall Effect Sensor/Z ==
  Electrical Reference1 : fl_lib/Electrical/Electrical Elements/Electrical Reference
  PS-Simulink Converter 2 : nesl_utility/PS-Simulink Converter  PhysicalDomain=network_engine_domain  SubClassName=ps_output  LeftPortType=input  RightPortType=output  PseudoPeriodic=off  Frequencies=[]  VectorFormat=1-D array  Unit=V  AffineConversion=off
  Voltage Sensor : fl_lib/Electrical/Electrical Sensors/Voltage Sensor
  Vz : Scope
  u : PMIOPort  Side=Left
  wires:
  PS-Simulink Converter 2/1 -> Vz/1
  connections:
  Voltage Sensor/RConn2 -- Electrical Reference1/LConn1
  Voltage Sensor/RConn1 -- PS-Simulink Converter 2/LConn1
  u/RConn1 -- Voltage Sensor/LConn1
